simulink model "ADIODEcontrol"  (Simulink 7.3)
settings: Solver=ode4  StartTime=0.0  StopTime=tof  FixedStep=dtSim  RelTol=1e-3
InitFcn:
  | initADIODEcontrol
StopFcn:
  | plotlab
values from neighbouring files (symbols this model uses):
  Arm = -2    [initADIODEcontrol.m]
  As = -10    [initADIODEcontrol.m]
  B = 1    [initADIODEcontrol.m]
  Brm = 2    [initADIODEcontrol.m]
  dtController = dtSim    (= 0.001)    [initADIODEcontrol.m]
  epsilon = 0.05    [initADIODEcontrol.m]
  epsilontheta = 0.1    [initADIODEcontrol.m]
  GammaW = 100    [initADIODEcontrol.m]
  lambdae2 = 10    [initADIODEcontrol.m]
  nofbasis = length(xis)*length(uis)    [initADIODEcontrol.m]
  Ps = lyap(As',Q)    [initADIODEcontrol.m]
  u0 = 0    [initADIODEcontrol.m]
  W0 = zeros(nofbasis,1)    [initADIODEcontrol.m]
  Wbound = 10    [initADIODEcontrol.m]
  x0 = [0 0]'    [initADIODEcontrol.m]
  xhat0 = 0    [initADIODEcontrol.m]
  xr0 = 0    [initADIODEcontrol.m]
  xu = zeros(nofbasis,2)    [initADIODEcontrol.m]
undefined symbols (not defined in the file or in its folder): DiscIntNeverNeededParam, Intmax, Intmin
libraries: dspbuff3 x3, vrlib x1, simulink x1
settings Model: Creator=Alp  LastModifiedBy=alpmarangoz
settings SolverCC: AutoInsertRateTranBlk=on

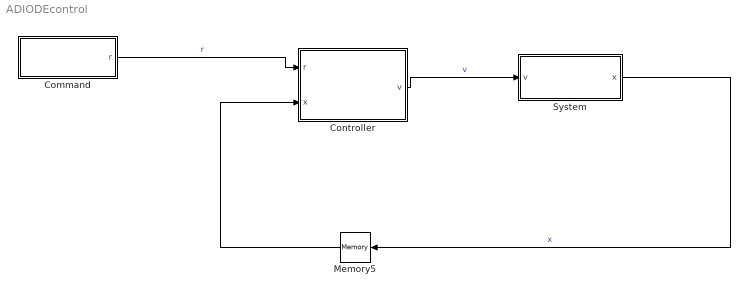
== system ADIODEcontrol ==
  Command : Subsystem  TreatAsAtomicUnit=on  SystemSampleTime=dtController
  Controller : Subsystem  TreatAsAtomicUnit=on  SystemSampleTime=dtController
  Memory5 : Memory  X0=xhat0  InheritSampleTime=on  LinearizeMemory=on  LinearizeAsDelay=on
  System : Subsystem  TreatAsAtomicUnit=on
  wires:
  Command/1(r) -> Controller/1(r)  "r"
  Controller/1(v) -> System/1(v)  "v"
  System/1(x) -> Memory5/1  "x"
  Memory5/1 -> Controller/2(x)

== system ADIODEcontrol/Command ==
  From Workspace : FromWorkspace  VariableName=rData  OutputAfterFinalValue=Setting to zero
  Reshape : Reshape  OutputDimensionality=Column vector (2-D)
  r : Outport
  wires:
  From Workspace/1 -> Reshape/1  "r"
  Reshape/1 -> r/1  "r"

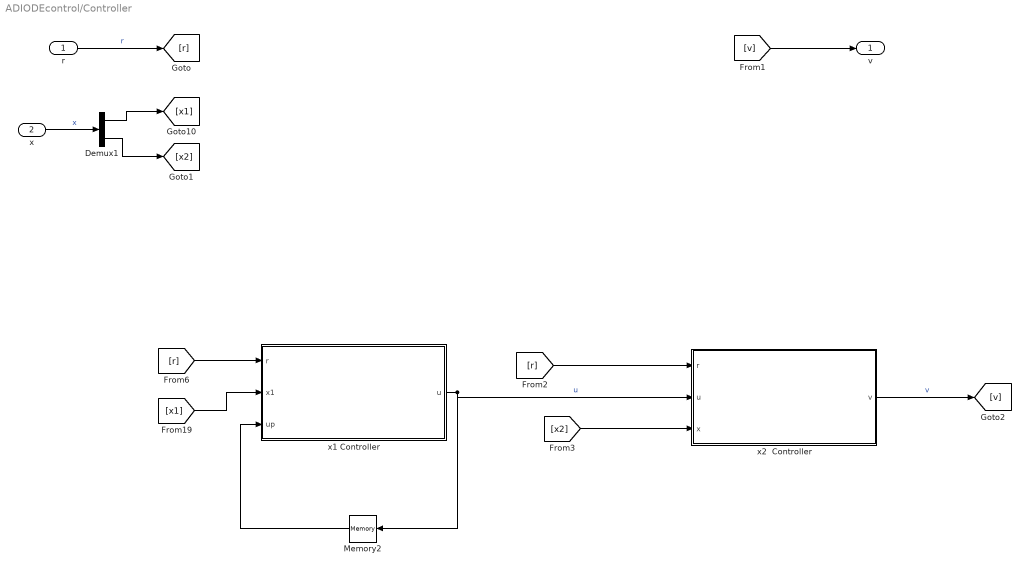
== system ADIODEcontrol/Controller ==
  r : Inport  OutDataType=fixdt(1, 16)  OutScaling=2^0
  x : Inport  Port=2  OutDataType=fixdt(1, 16)  OutScaling=2^0
  Demux1 : Demux  Outputs=2
  Memory2 : Memory  X0=u0  InheritSampleTime=on  LinearizeMemory=on  LinearizeAsDelay=on
  x1 Controller : Subsystem  TreatAsAtomicUnit=on  SystemSampleTime=dtController
  x2  Controller : Subsystem  TreatAsAtomicUnit=on  SystemSampleTime=dtController
  v : Outport  OutDataType=fixdt(1, 16)  OutScaling=2^0
  wires:
  r/1 -> [r]  "r"
  [v] -> v/1
  Demux1/1 -> [x1]
  Demux1/2 -> [x2]
  x/1 -> Demux1/1  "x"
  [r] -> x1 Controller/1(r)
  [x1] -> x1 Controller/2(x1)
  x1 Controller/1(u) -> Memory2/1, x2  Controller/2(u)  "u"
  Memory2/1 -> x1 Controller/3(up)
  [r] -> x2  Controller/1(r)
  [x2] -> x2  Controller/3(x)
  x2  Controller/1(v) -> [v]  "v"

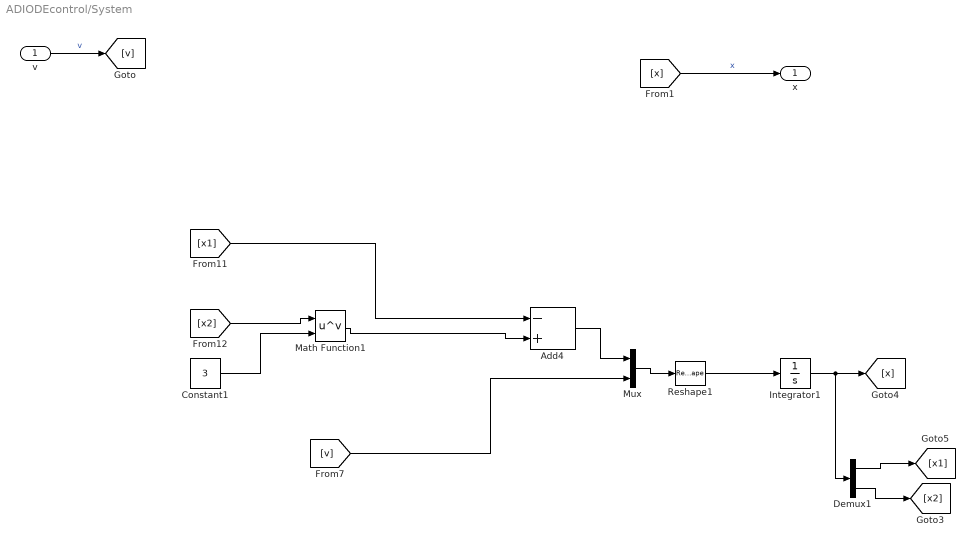
== system ADIODEcontrol/System ==
  v : Inport  OutDataType=fixdt(1, 16)  OutScaling=2^0
  Add4 : Sum  Inputs=-+  OutDataType=fixdt(1, 16)  OutScaling=2^-10
  Constant1 : Constant  Value=3  OutDataType=fixdt(1, 16)  OutScaling=2^0
  Demux1 : Demux  Outputs=2
  Integrator1 : Integrator  InitialCondition=x0
  Math Function1 : Math  Operator=pow  OutDataType=fixdt(1, 16)  OutScaling=2^0  SaturateOnIntegerOverflow=on
  Mux : Mux  Inputs=2
  Reshape1 : Reshape  OutputDimensionality=Column vector (2-D)
  x : Outport  OutDataType=fixdt(1, 16)  OutScaling=2^0
  wires:
  v/1 -> [v]  "v"
  [x] -> x/1  "x"
  [x2] -> Math Function1/1
  Constant1/1 -> Math Function1/2
  [x1] -> Add4/1
  Math Function1/1 -> Add4/2
  Integrator1/1 -> [x], Demux1/1
  Add4/1 -> Mux/1
  [v] -> Mux/2
  Mux/1 -> Reshape1/1
  Reshape1/1 -> Integrator1/1
  Demux1/1 -> [x1]
  Demux1/2 -> [x2]

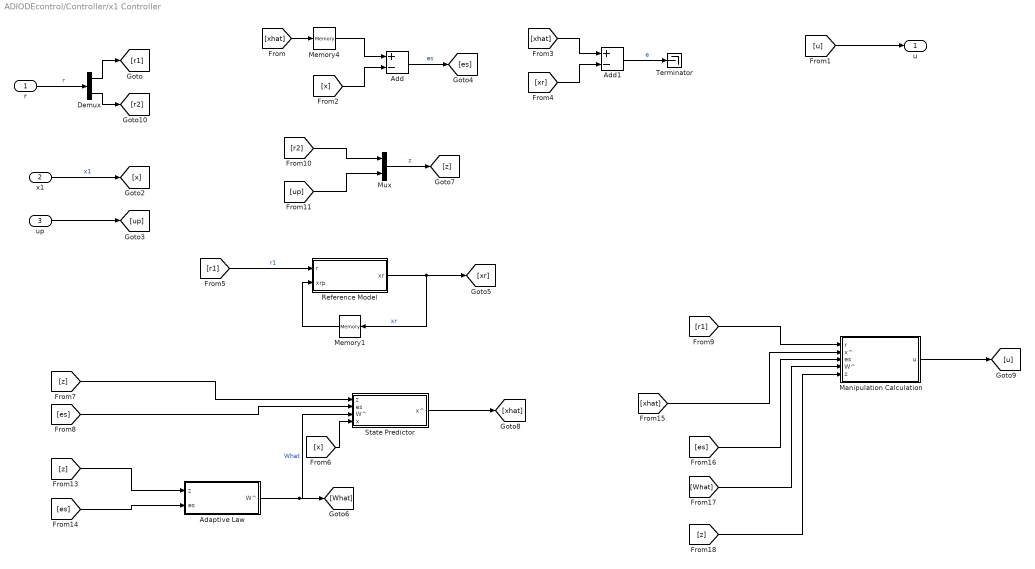
== system ADIODEcontrol/Controller/x1 Controller ==
  r : Inport  OutDataType=fixdt(1, 16)  OutScaling=2^0
  x1 : Inport  Port=2  OutDataType=fixdt(1, 16)  OutScaling=2^0
  up : Inport  Port=3  OutDataType=fixdt(1, 16)  OutScaling=2^0
  Adaptive Law : Subsystem  TreatAsAtomicUnit=on
  Add : Sum  Inputs=+-  OutDataType=fixdt(1, 16)  OutScaling=2^-10
  Add1 : Sum  Inputs=+-  OutDataType=fixdt(1, 16)  OutScaling=2^-10
  Demux : Demux  Outputs=2
  Manipulation Calculation : Subsystem  TreatAsAtomicUnit=on
  Memory1 : Memory  X0=xr0  InheritSampleTime=on  LinearizeMemory=on  LinearizeAsDelay=on
  Memory4 : Memory  X0=xhat0  InheritSampleTime=on  LinearizeMemory=on  LinearizeAsDelay=on
  Mux : Mux  Inputs=2
  Reference Model : Subsystem  TreatAsAtomicUnit=on
  State Predictor : Subsystem  TreatAsAtomicUnit=on
  Terminator : Terminator
  u : Outport  OutDataType=fixdt(1, 16)  OutScaling=2^0
  wires:
  [u] -> u/1
  x1/1 -> [x]  "x1"
  up/1 -> [up]
  [xhat] -> Memory4/1
  [x] -> Add/2
  [xhat] -> Add1/1
  [xr] -> Add1/2
  Add/1 -> [es]  "es"
  Add1/1 -> Terminator/1  "e"
  Reference Model/1(xr) -> [xr], Memory1/1  "xr"
  [r1] -> Reference Model/1(r)  "r1"
  Memory4/1 -> Add/1
  [z] -> Adaptive Law/1(z)
  [es] -> Adaptive Law/2(es)
  Adaptive Law/1(W^) -> State Predictor/3(W^), [What]  "What"
  [z] -> State Predictor/1(z)
  [es] -> State Predictor/2(es)
  State Predictor/1(x^) -> [xhat]
  [r1] -> Manipulation Calculation/1(r)
  [xhat] -> Manipulation Calculation/2(x^)
  [es] -> Manipulation Calculation/3(es)
  [What] -> Manipulation Calculation/4(W^)
  [z] -> Manipulation Calculation/5(z)
  Manipulation Calculation/1(u) -> [u]
  Memory1/1 -> Reference Model/2(xrp)
  [r2] -> Mux/1
  [up] -> Mux/2
  Mux/1 -> [z]  "z"
  [x] -> State Predictor/4(x)
  r/1 -> Demux/1  "r"
  Demux/1 -> [r1]
  Demux/2 -> [r2]

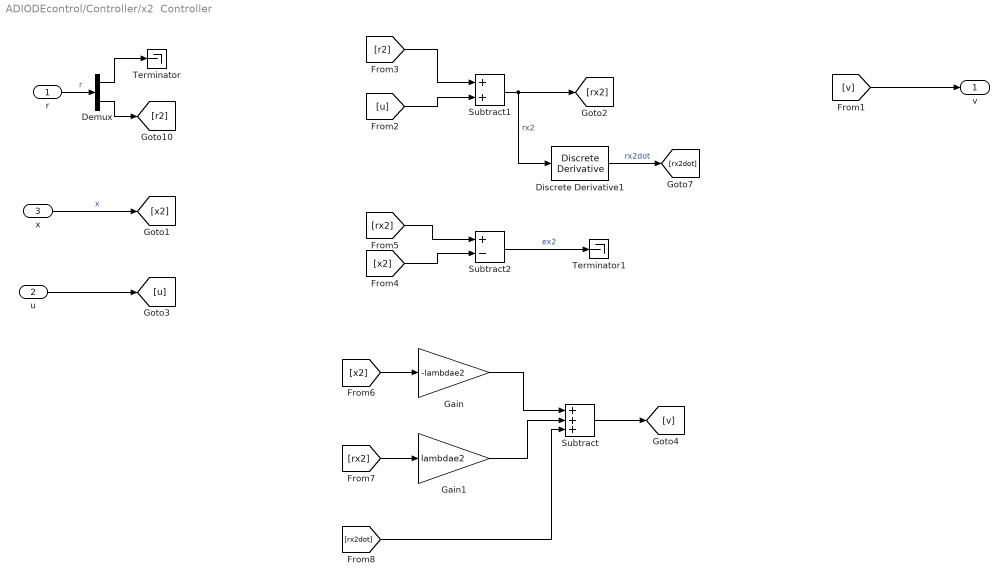
== system ADIODEcontrol/Controller/x2  Controller ==
  r : Inport  OutDataType=fixdt(1, 16)  OutScaling=2^0
  u : Inport  Port=2  OutDataType=fixdt(1, 16)  OutScaling=2^0
  x : Inport  Port=3  OutDataType=fixdt(1, 16)  OutScaling=2^0
  Demux : Demux  Outputs=2
  Discrete Derivative1 : simulink/Discrete/Discrete Derivative  SystemSampleTime=-1  gainval=1.0  ICPrevScaledInput=0.0  OutMin=[]  OutMax=[]  OutDataType=fixdt(1, 16)  OutScaling=2^-10  DoSatur=off
  Gain : Gain  Gain=-lambdae2  ParameterDataType=fixdt(1, 16)  ParameterScaling=2^0  OutDataType=fixdt(1, 16)  OutScaling=2^0
  Gain1 : Gain  Gain=lambdae2  ParameterDataType=fixdt(1, 16)  ParameterScaling=2^0  OutDataType=fixdt(1, 16)  OutScaling=2^0
  Subtract : Sum  Inputs=+++  OutDataType=fixdt(1, 16)  OutScaling=2^-10
  Subtract1 : Sum  OutDataType=fixdt(1, 16)  OutScaling=2^-10
  Subtract2 : Sum  Inputs=+-  OutDataType=fixdt(1, 16)  OutScaling=2^-10
  Terminator : Terminator
  Terminator1 : Terminator
  v : Outport  OutDataType=fixdt(1, 16)  OutScaling=2^0
  wires:
  Demux/2 -> [r2]
  Demux/1 -> Terminator/1
  r/1 -> Demux/1  "r"
  u/1 -> [u]
  [v] -> v/1
  x/1 -> [x2]  "x"
  [x2] -> Gain/1
  [rx2] -> Gain1/1
  Gain/1 -> Subtract/1
  Gain1/1 -> Subtract/2
  [r2] -> Subtract1/1
  [u] -> Subtract1/2
  Subtract1/1 -> [rx2], Discrete Derivative1/1  "rx2"
  Subtract/1 -> [v]
  [x2] -> Subtract2/2
  Subtract2/1 -> Terminator1/1  "ex2"
  [rx2] -> Subtract2/1
  Discrete Derivative1/1 -> [rx2dot]  "rx2dot"
  [rx2dot] -> Subtract/3

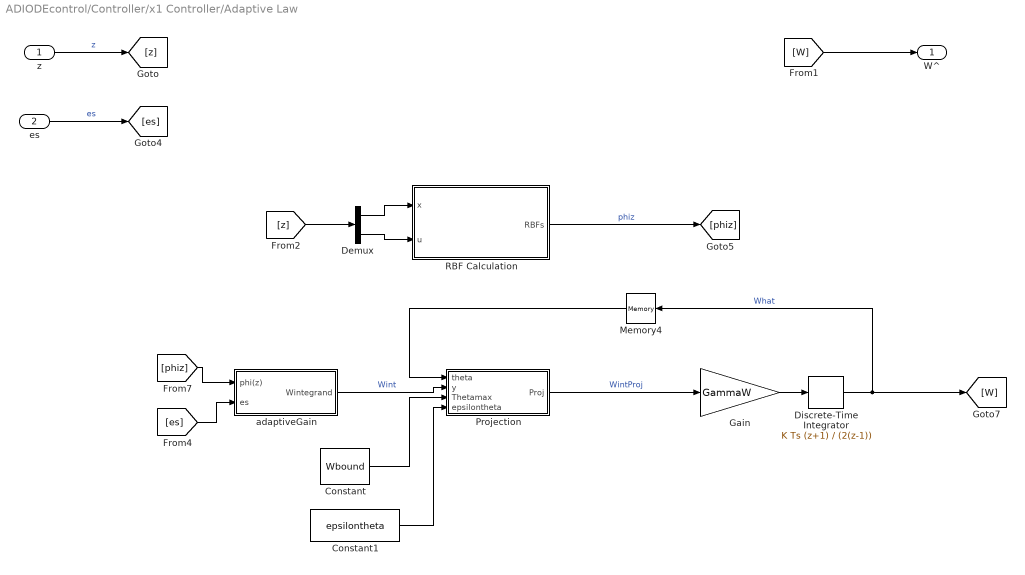
== system ADIODEcontrol/Controller/x1 Controller/Adaptive Law ==
  z : Inport  OutDataType=fixdt(1, 16)  OutScaling=2^0
  es : Inport  Port=2  OutDataType=fixdt(1, 16)  OutScaling=2^0
  Constant : Constant  Value=Wbound  OutDataType=fixdt(1, 16)  OutScaling=2^0
  Constant1 : Constant  Value=epsilontheta  OutDataType=fixdt(1, 16)  OutScaling=2^0
  Demux : Demux  Outputs=2
  Discrete-Time Integrator : DiscreteIntegrator  IntegratorMethod=Integration: Trapezoidal  InitialCondition=W0  SampleTime=-1  OutDataType=fixdt(1, 16)  OutScaling=2^0  LimitOutput=on  UpperSaturationLimit=Wbound  LowerSaturationLimit=-Wbound  ICPrevOutput=DiscIntNeverNeededParam  ICPrevScaledInput=DiscIntNeverNeededParam
  Gain : Gain  Gain=GammaW  ParameterDataType=fixdt(1, 16)  ParameterScaling=2^0  OutDataType=fixdt(1, 16)  OutScaling=2^0
  Memory4 : Memory  X0=W0  InheritSampleTime=on  LinearizeMemory=on  LinearizeAsDelay=on
  Projection : Subsystem  TreatAsAtomicUnit=on
  RBF Calculation : Subsystem  TreatAsAtomicUnit=on
  adaptiveGain : Subsystem  TreatAsAtomicUnit=on
  W^ : Outport  OutDataType=fixdt(1, 16)  OutScaling=2^0
  wires:
  z/1 -> [z]  "z"
  es/1 -> [es]  "es"
  [es] -> adaptiveGain/2(es)
  [phiz] -> adaptiveGain/1(phi(z))
  [W] -> W^/1
  Discrete-Time Integrator/1 -> [W], Memory4/1  "What"
  Gain/1 -> Discrete-Time Integrator/1
  RBF Calculation/1(RBFs) -> [phiz]  "phiz"
  [z] -> Demux/1
  Demux/1 -> RBF Calculation/1(x)
  Demux/2 -> RBF Calculation/2(u)
  Projection/1(Proj) -> Gain/1  "WintProj"
  adaptiveGain/1(Wintegrand) -> Projection/2(y)  "Wint"
  Memory4/1 -> Projection/1(theta)
  Constant/1 -> Projection/3(Thetamax)
  Constant1/1 -> Projection/4(epsilontheta)

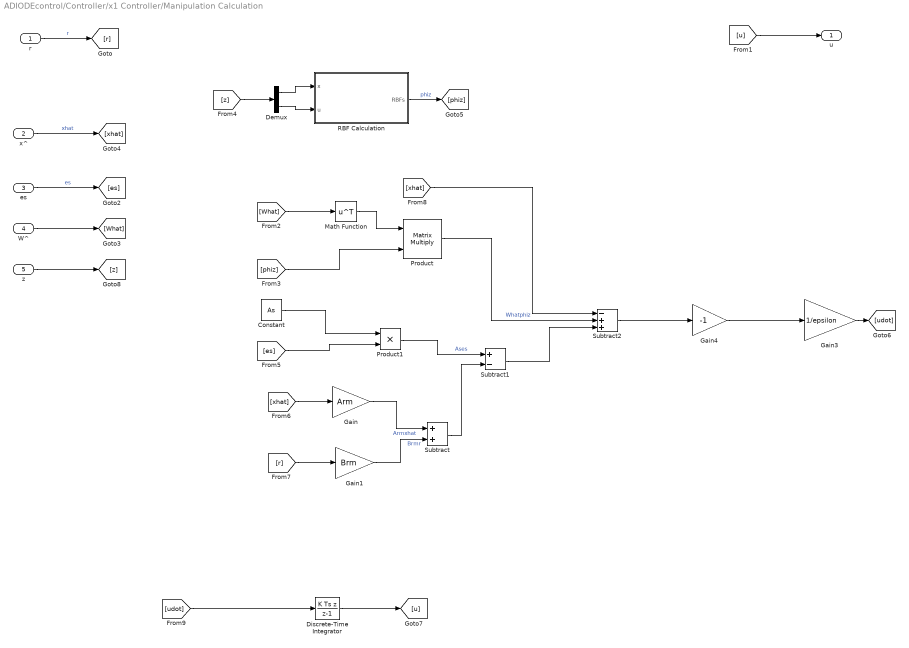
== system ADIODEcontrol/Controller/x1 Controller/Manipulation Calculation ==
  r : Inport  OutDataType=fixdt(1, 16)  OutScaling=2^0
  x^ : Inport  Port=2  OutDataType=fixdt(1, 16)  OutScaling=2^0
  es : Inport  Port=3  OutDataType=fixdt(1, 16)  OutScaling=2^0
  W^ : Inport  Port=4  OutDataType=fixdt(1, 16)  OutScaling=2^0
  z : Inport  Port=5  OutDataType=fixdt(1, 16)  OutScaling=2^0
  Constant : Constant  Value=As  OutDataType=fixdt(1, 16)  OutScaling=2^0
  Demux : Demux  Outputs=2
  Discrete-Time Integrator : DiscreteIntegrator  IntegratorMethod=Integration: Backward Euler  InitialCondition=u0  InitialConditionMode=State only (most efficient)  SampleTime=-1  OutDataType=fixdt(1, 16)  OutScaling=2^0  UpperSaturationLimit=Intmax  LowerSaturationLimit=Intmin  ICPrevOutput=DiscIntNeverNeededParam  ICPrevScaledInput=DiscIntNeverNeededParam
  Gain : Gain  Gain=Arm  ParameterDataType=fixdt(1, 16)  ParameterScaling=2^0  OutDataType=fixdt(1, 16)  OutScaling=2^0
  Gain1 : Gain  Gain=Brm  ParameterDataType=fixdt(1, 16)  ParameterScaling=2^0  OutDataType=fixdt(1, 16)  OutScaling=2^0
  Gain3 : Gain  Gain=1/epsilon  ParameterDataType=fixdt(1, 16)  ParameterScaling=2^0  OutDataType=fixdt(1, 16)  OutScaling=2^0
  Gain4 : Gain  Gain=-1  ParameterDataType=fixdt(1, 16)  ParameterScaling=2^0  OutDataType=fixdt(1, 16)  OutScaling=2^0
  Math Function : Math  Operator=transpose  OutDataType=fixdt(1, 16)  OutScaling=2^0  SaturateOnIntegerOverflow=on
  Product : Product  Multiplication=Matrix(*)  OutDataType=fixdt(1, 16)  OutScaling=2^0  RndMeth=Zero
  Product1 : Product  OutDataType=fixdt(1, 16)  OutScaling=2^0  RndMeth=Zero
  RBF Calculation : Subsystem  TreatAsAtomicUnit=on
  Subtract : Sum  OutDataType=fixdt(1, 16)  OutScaling=2^-10
  Subtract1 : Sum  Inputs=+-  OutDataType=fixdt(1, 16)  OutScaling=2^-10
  Subtract2 : Sum  Inputs=-++  OutDataType=fixdt(1, 16)  OutScaling=2^-10
  u : Outport  OutDataType=fixdt(1, 16)  OutScaling=2^0
  wires:
  r/1 -> [r]  "r"
  [u] -> u/1
  x^/1 -> [xhat]  "xhat"
  es/1 -> [es]  "es"
  W^/1 -> [What]
  [What] -> Math Function/1
  Math Function/1 -> Product/1
  [phiz] -> Product/2
  Constant/1 -> Product1/1
  [xhat] -> Gain/1
  [r] -> Gain1/1
  Gain3/1 -> [udot]
  z/1 -> [z]
  [es] -> Product1/2
  RBF Calculation/1(RBFs) -> [phiz]  "phiz"
  [z] -> Demux/1
  Demux/1 -> RBF Calculation/1(x)
  Demux/2 -> RBF Calculation/2(u)
  [udot] -> Discrete-Time Integrator/1
  Discrete-Time Integrator/1 -> [u]
  Gain4/1 -> Gain3/1
  Gain/1 -> Subtract/1  "Armxhat"
  Gain1/1 -> Subtract/2  "Brmr"
  Product1/1 -> Subtract1/1  "Ases"
  Subtract/1 -> Subtract1/2
  Subtract2/1 -> Gain4/1
  [xhat] -> Subtract2/1
  Product/1 -> Subtract2/2  "Whatphiz"
  Subtract1/1 -> Subtract2/3

== system ADIODEcontrol/Controller/x1 Controller/Reference Model ==
  r : Inport  OutDataType=fixdt(1, 16)  OutScaling=2^0
  xrp : Inport  Port=2  OutDataType=fixdt(1, 16)  OutScaling=2^0
  Add1 : Sum  OutDataType=fixdt(1, 16)  OutScaling=2^-10
  Discrete-Time Integrator : DiscreteIntegrator  IntegratorMethod=Integration: Backward Euler  InitialCondition=xr0  InitialConditionMode=State only (most efficient)  SampleTime=-1  OutDataType=fixdt(1, 16)  OutScaling=2^0  UpperSaturationLimit=Intmax  LowerSaturationLimit=Intmin  ICPrevOutput=DiscIntNeverNeededParam  ICPrevScaledInput=DiscIntNeverNeededParam
  Gain1 : Gain  Gain=Arm  Multiplication=Matrix(K*u)  ParameterDataType=fixdt(1, 16)  ParameterScaling=2^0  OutDataType=fixdt(1, 16)  OutScaling=2^0
  Gain2 : Gain  Gain=Brm  Multiplication=Matrix(K*u)  ParameterDataType=fixdt(1, 16)  ParameterScaling=2^0  OutDataType=fixdt(1, 16)  OutScaling=2^0
  Reshape : Reshape  OutputDimensionality=Column vector (2-D)
  xr : Outport  OutDataType=fixdt(1, 16)  OutScaling=2^0
  wires:
  [xrp] -> Gain1/1
  r/1 -> [u]  "r"
  [u] -> Gain2/1
  Gain1/1 -> Add1/1
  Gain2/1 -> Add1/2
  Add1/1 -> Reshape/1  "xrmdot"
  Reshape/1 -> Discrete-Time Integrator/1
  Discrete-Time Integrator/1 -> xr/1  "xr"
  xrp/1 -> [xrp]

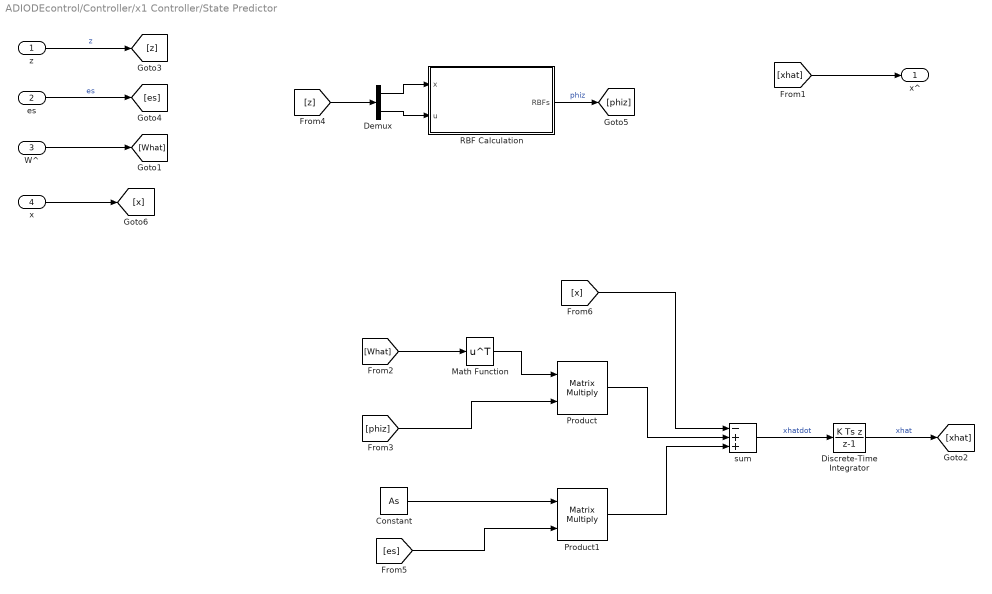
== system ADIODEcontrol/Controller/x1 Controller/State Predictor ==
  z : Inport  OutDataType=fixdt(1, 16)  OutScaling=2^0
  es : Inport  Port=2  OutDataType=fixdt(1, 16)  OutScaling=2^0
  W^ : Inport  Port=3  OutDataType=fixdt(1, 16)  OutScaling=2^0
  x : Inport  Port=4  OutDataType=fixdt(1, 16)  OutScaling=2^0
  Constant : Constant  Value=As  OutDataType=fixdt(1, 16)  OutScaling=2^0
  Demux : Demux  Outputs=2
  Discrete-Time Integrator : DiscreteIntegrator  IntegratorMethod=Integration: Backward Euler  InitialCondition=xhat0  InitialConditionMode=State only (most efficient)  SampleTime=-1  OutDataType=fixdt(1, 16)  OutScaling=2^0  UpperSaturationLimit=Intmax  LowerSaturationLimit=Intmin  ICPrevOutput=DiscIntNeverNeededParam  ICPrevScaledInput=DiscIntNeverNeededParam
  Math Function : Math  Operator=transpose  OutDataType=fixdt(1, 16)  OutScaling=2^0  SaturateOnIntegerOverflow=on
  Product : Product  Multiplication=Matrix(*)  OutDataType=fixdt(1, 16)  OutScaling=2^0  RndMeth=Zero
  Product1 : Product  Multiplication=Matrix(*)  OutDataType=fixdt(1, 16)  OutScaling=2^0  RndMeth=Zero
  RBF Calculation : Subsystem  TreatAsAtomicUnit=on
  sum : Sum  Inputs=-++  OutDataType=fixdt(1, 16)  OutScaling=2^-10
  x^ : Outport  OutDataType=fixdt(1, 16)  OutScaling=2^0
  wires:
  W^/1 -> [What]
  es/1 -> [es]  "es"
  [What] -> Math Function/1
  Math Function/1 -> Product/1
  [phiz] -> Product/2
  Constant/1 -> Product1/1
  [es] -> Product1/2
  sum/1 -> Discrete-Time Integrator/1  "xhatdot"
  Discrete-Time Integrator/1 -> [xhat]  "xhat"
  z/1 -> [z]  "z"
  [xhat] -> x^/1
  RBF Calculation/1(RBFs) -> [phiz]  "phiz"
  [z] -> Demux/1
  Demux/1 -> RBF Calculation/1(x)
  Demux/2 -> RBF Calculation/2(u)
  x/1 -> [x]
  [x] -> sum/1
  Product/1 -> sum/2
  Product1/1 -> sum/3

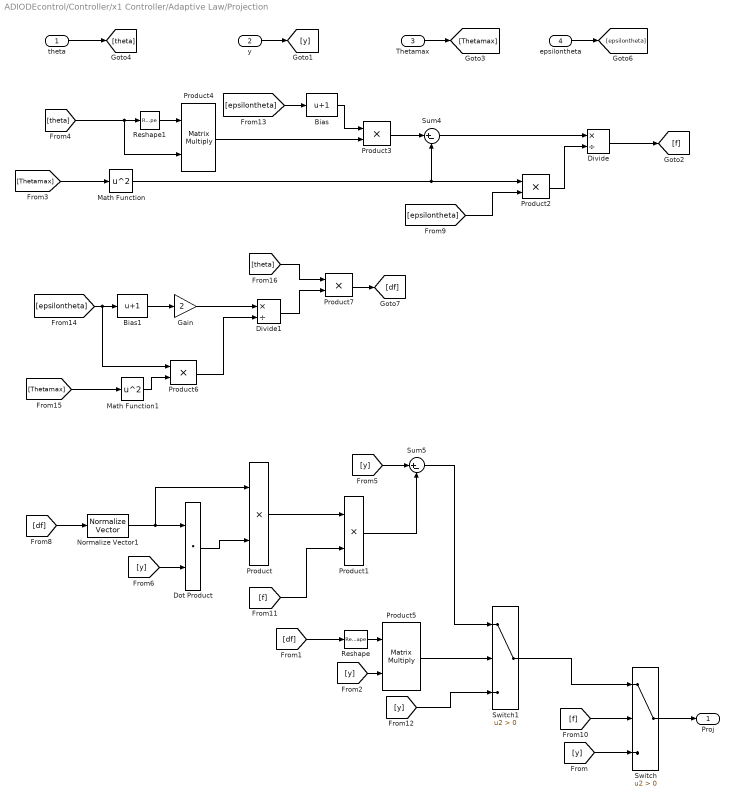
== system ADIODEcontrol/Controller/x1 Controller/Adaptive Law/Projection ==
  theta : Inport  OutDataType=sfix(16)  OutScaling=2^0
  y : Inport  Port=2  OutDataType=sfix(16)  OutScaling=2^0
  Thetamax : Inport  Port=3  OutDataType=sfix(16)  OutScaling=2^0
  epsilontheta : Inport  Port=4  OutDataType=sfix(16)  OutScaling=2^0
  Bias : Bias  Bias=1
  Bias1 : Bias  Bias=1
  Divide : Product  Inputs=*/  OutDataType=fixdt(1, 16)  OutScaling=2^-10
  Divide1 : Product  Inputs=*/  OutDataType=fixdt(1, 16)  OutScaling=2^-10
  Dot Product : DotProduct  OutDataType=fixdt(1, 16)  OutScaling=2^-10  InputSameDT=on  OutDataTypeStr=Inherit: Inherit via internal rule
  Gain : Gain  Gain=2  ParameterDataType=fixdt(1, 16)  ParameterScaling=2^0  OutDataType=fixdt(1, 16)  OutScaling=2^0
  Math Function : Math  Operator=square  OutDataType=fixdt(1, 16)  OutScaling=2^0  SaturateOnIntegerOverflow=on
  Math Function1 : Math  Operator=square  OutDataType=fixdt(1, 16)  OutScaling=2^0  SaturateOnIntegerOverflow=on
  Normalize Vector1 : vrlib/Utilities/Normalize Vector  SystemSampleTime=-1  maxzero=0
  Product{,1..3,6..7} (6 alike) : Product  OutDataType=fixdt(1, 16)  OutScaling=2^0  RndMeth=Zero
  Product4 : Product  Multiplication=Matrix(*)  OutDataType=sfix(16)  OutScaling=2^0  RndMeth=Zero
  Product5 : Product  Multiplication=Matrix(*)  OutDataType=sfix(16)  OutScaling=2^0  RndMeth=Zero
  Reshape : Reshape  OutputDimensionality=Row vector (2-D)
  Reshape1 : Reshape  OutputDimensionality=Row vector (2-D)
  Sum4 : Sum  Inputs=|+-  OutDataType=sfix(16)  OutScaling=2^0
  Sum5 : Sum  Inputs=|+-  OutDataType=sfix(16)  OutScaling=2^0
  Switch : Switch  Criteria=u2 > Threshold  OutDataType=sfix(16)  OutScaling=2^0
  Switch1 : Switch  Criteria=u2 > Threshold  OutDataType=sfix(16)  OutScaling=2^0
  Proj : Outport  OutDataType=sfix(16)  OutScaling=2^0
  wires:
  [f] -> Switch/2
  y/1 -> [y]
  Switch/1 -> Proj/1
  Product5/1 -> Switch1/2
  [y] -> Product5/2
  Sum4/1 -> Divide/1
  Math Function/1 -> Sum4/2, Product2/1
  Product4/1 -> Product3/2
  [theta] -> Reshape1/1, Product4/2
  [df] -> Reshape/1
  Reshape/1 -> Product5/1
  Reshape1/1 -> Product4/1
  theta/1 -> [theta]
  [y] -> Switch/3
  Switch1/1 -> Switch/1
  [y] -> Sum5/1
  Product/1 -> Product1/1
  [y] -> Switch1/3
  Product1/1 -> Sum5/2
  Sum5/1 -> Switch1/1
  [f] -> Product1/2
  [df] -> Normalize Vector1/1
  Normalize Vector1/1 -> Dot Product/1, Product/1
  [y] -> Dot Product/2
  Dot Product/1 -> Product/2
  Thetamax/1 -> [Thetamax]
  [Thetamax] -> Math Function/1
  epsilontheta/1 -> [epsilontheta]
  [epsilontheta] -> Product2/2
  Product2/1 -> Divide/2
  Divide/1 -> [f]
  Product3/1 -> Sum4/1
  Bias/1 -> Product3/1
  [epsilontheta] -> Bias/1
  [epsilontheta] -> Bias1/1, Product6/1
  Bias1/1 -> Gain/1
  Gain/1 -> Divide1/1
  [Thetamax] -> Math Function1/1
  Math Function1/1 -> Product6/2
  Product6/1 -> Divide1/2
  Product7/1 -> [df]
  [theta] -> Product7/1
  Divide1/1 -> Product7/2

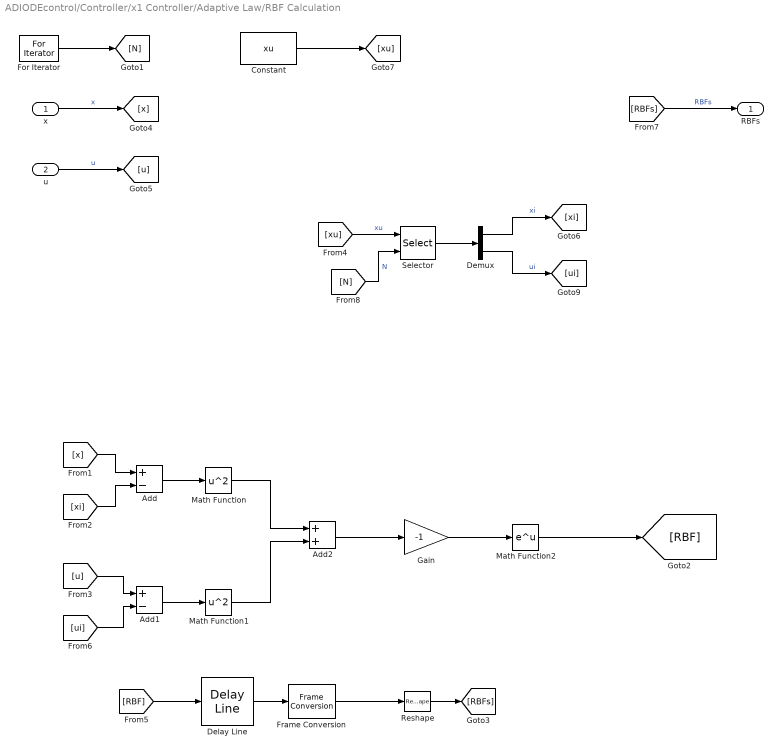
== system ADIODEcontrol/Controller/x1 Controller/Adaptive Law/RBF Calculation ==
  x : Inport  OutDataType=fixdt(1, 16)  OutScaling=2^0
  u : Inport  Port=2  OutDataType=fixdt(1, 16)  OutScaling=2^0
  Add : Sum  Inputs=+-  OutDataType=fixdt(1, 16)  OutScaling=2^-10
  Add1 : Sum  Inputs=+-  OutDataType=fixdt(1, 16)  OutScaling=2^-10
  Add2 : Sum  OutDataType=fixdt(1, 16)  OutScaling=2^-10
  Constant : Constant  Value=xu  VectorParams1D=off  OutDataType=fixdt(1, 16)  OutScaling=2^0
  Delay Line : dspbuff3/Delay Line  siz=nofbasis  ic=zeros(nofbasis,1)  directfeed=on  enable_output=off  hold_output=off
  Demux : Demux  Outputs=2
  For Iterator : ForIterator  IterationLimit=nofbasis
  Frame Conversion : FrameConversion  OutFrame=Sample-based
  Gain : Gain  Gain=-1  ParameterDataType=fixdt(1, 16)  ParameterScaling=2^0  OutDataType=fixdt(1, 16)  OutScaling=2^0
  Math Function : Math  Operator=square  OutDataType=fixdt(1, 16)  OutScaling=2^0  SaturateOnIntegerOverflow=on
  Math Function1 : Math  Operator=square  OutDataType=fixdt(1, 16)  OutScaling=2^0  SaturateOnIntegerOverflow=on
  Math Function2 : Math  OutDataType=fixdt(1, 16)  OutScaling=2^0  SaturateOnIntegerOverflow=on
  Reshape : Reshape  OutputDimensionality=Column vector (2-D)
  Selector : Selector  NumberOfDimensions=2  IndexOptions=Index vector (port),Select all  Indices=[1 3],1  OutputSizes=1,1
  RBFs : Outport  OutDataType=fixdt(1, 16)  OutScaling=2^0
  wires:
  For Iterator/1 -> [N]
  [RBF] -> Delay Line/1
  Delay Line/1 -> Frame Conversion/1
  [RBFs] -> RBFs/1  "RBFs"
  Frame Conversion/1 -> Reshape/1
  x/1 -> [x]  "x"
  u/1 -> [u]  "u"
  [xu] -> Selector/1  "xu"
  [N] -> Selector/2  "N"
  [x] -> Add/1
  [xi] -> Add/2
  Add/1 -> Math Function/1
  [u] -> Add1/1
  [ui] -> Add1/2
  Add1/1 -> Math Function1/1
  Math Function/1 -> Add2/1
  Math Function1/1 -> Add2/2
  Add2/1 -> Gain/1
  Gain/1 -> Math Function2/1
  Math Function2/1 -> [RBF]
  Reshape/1 -> [RBFs]
  Constant/1 -> [xu]
  Selector/1 -> Demux/1
  Demux/1 -> [xi]  "xi"
  Demux/2 -> [ui]  "ui"

== system ADIODEcontrol/Controller/x1 Controller/Adaptive Law/adaptiveGain ==
  phi(z) : Inport  OutDataType=fixdt(1, 16)  OutScaling=2^0
  es : Inport  Port=2  OutDataType=fixdt(1, 16)  OutScaling=2^0
  Gain1 : Gain  Gain=-1  ParameterDataType=fixdt(1, 16)  ParameterScaling=2^0  OutDataType=fixdt(1, 16)  OutScaling=2^0
  Math Function : Math  Operator=transpose  OutDataType=sfix(16)  OutScaling=2^0  SaturateOnIntegerOverflow=on
  P : Constant  Value=Ps  VectorParams1D=off  OutDataType=fixdt(1, 16)  OutScaling=2^0
  Product1 : Product  Multiplication=Matrix(*)  OutDataType=fixdt(1, 16)  OutScaling=2^0  RndMeth=Zero
  Product3 : Product  Multiplication=Matrix(*)  OutDataType=fixdt(1, 16)  OutScaling=2^0  RndMeth=Zero
  Product5 : Product  Multiplication=Matrix(*)  OutDataType=fixdt(1, 16)  OutScaling=2^0  RndMeth=Zero
  b : Constant  Value=B  VectorParams1D=off  OutDataType=fixdt(1, 16)  OutScaling=2^0
  Wintegrand : Outport  OutDataType=fixdt(1, 16)  OutScaling=2^0
  wires:
  P/1 -> Product5/1
  b/1 -> Product5/2
  es/1 -> Math Function/1
  Math Function/1 -> Product1/1
  Product5/1 -> Product1/2
  phi(z)/1 -> Gain1/1
  Product1/1 -> Product3/2
  Product3/1 -> Wintegrand/1
  Gain1/1 -> Product3/1

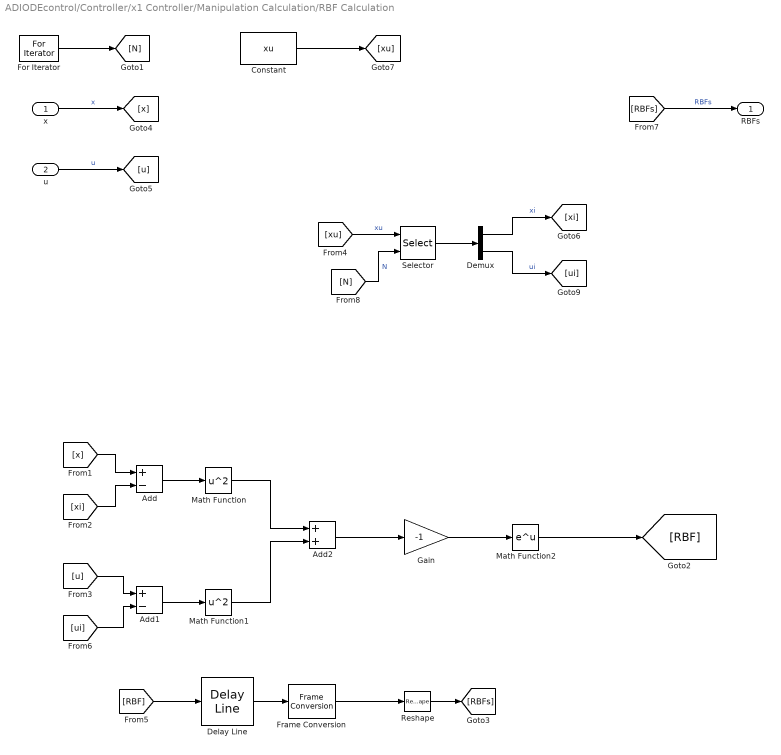
== system ADIODEcontrol/Controller/x1 Controller/Manipulation Calculation/RBF Calculation ==
  x : Inport  OutDataType=fixdt(1, 16)  OutScaling=2^0
  u : Inport  Port=2  OutDataType=fixdt(1, 16)  OutScaling=2^0
  Add : Sum  Inputs=+-  OutDataType=fixdt(1, 16)  OutScaling=2^-10
  Add1 : Sum  Inputs=+-  OutDataType=fixdt(1, 16)  OutScaling=2^-10
  Add2 : Sum  OutDataType=fixdt(1, 16)  OutScaling=2^-10
  Constant : Constant  Value=xu  VectorParams1D=off  OutDataType=fixdt(1, 16)  OutScaling=2^0
  Delay Line : dspbuff3/Delay Line  siz=nofbasis  ic=zeros(nofbasis,1)  directfeed=on  enable_output=off  hold_output=off
  Demux : Demux  Outputs=2
  For Iterator : ForIterator  IterationLimit=nofbasis
  Frame Conversion : FrameConversion  OutFrame=Sample-based
  Gain : Gain  Gain=-1  ParameterDataType=fixdt(1, 16)  ParameterScaling=2^0  OutDataType=fixdt(1, 16)  OutScaling=2^0
  Math Function : Math  Operator=square  OutDataType=fixdt(1, 16)  OutScaling=2^0  SaturateOnIntegerOverflow=on
  Math Function1 : Math  Operator=square  OutDataType=fixdt(1, 16)  OutScaling=2^0  SaturateOnIntegerOverflow=on
  Math Function2 : Math  OutDataType=fixdt(1, 16)  OutScaling=2^0  SaturateOnIntegerOverflow=on
  Reshape : Reshape  OutputDimensionality=Column vector (2-D)
  Selector : Selector  NumberOfDimensions=2  IndexOptions=Index vector (port),Select all  Indices=[1 3],1  OutputSizes=1,1
  RBFs : Outport  OutDataType=fixdt(1, 16)  OutScaling=2^0
  wires:
  For Iterator/1 -> [N]
  [RBF] -> Delay Line/1
  Delay Line/1 -> Frame Conversion/1
  [RBFs] -> RBFs/1  "RBFs"
  Frame Conversion/1 -> Reshape/1
  x/1 -> [x]  "x"
  u/1 -> [u]  "u"
  [xu] -> Selector/1  "xu"
  [N] -> Selector/2  "N"
  [x] -> Add/1
  [xi] -> Add/2
  Add/1 -> Math Function/1
  [u] -> Add1/1
  [ui] -> Add1/2
  Add1/1 -> Math Function1/1
  Math Function/1 -> Add2/1
  Math Function1/1 -> Add2/2
  Add2/1 -> Gain/1
  Gain/1 -> Math Function2/1
  Math Function2/1 -> [RBF]
  Reshape/1 -> [RBFs]
  Constant/1 -> [xu]
  Selector/1 -> Demux/1
  Demux/1 -> [xi]  "xi"
  Demux/2 -> [ui]  "ui"

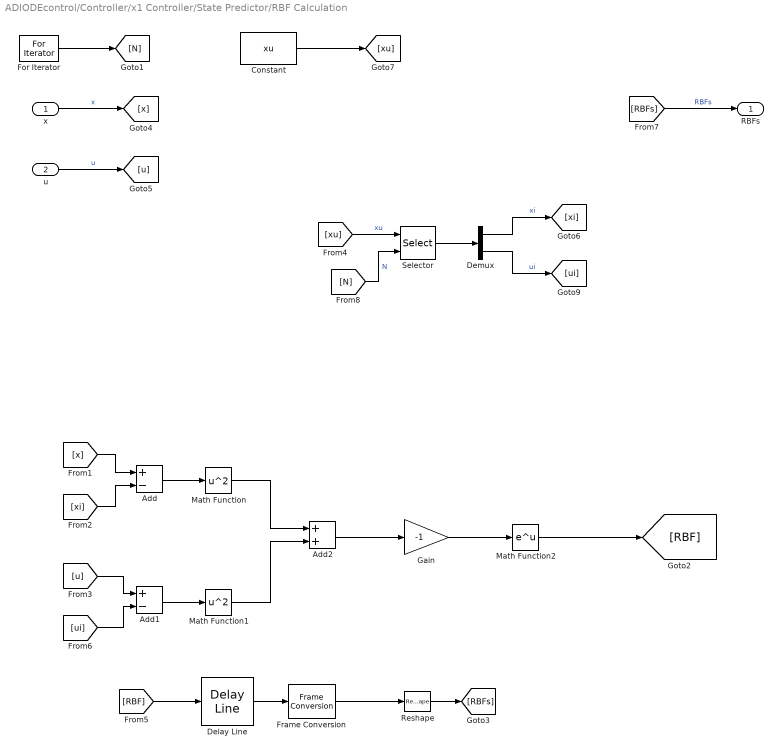
== system ADIODEcontrol/Controller/x1 Controller/State Predictor/RBF Calculation ==
  x : Inport  OutDataType=fixdt(1, 16)  OutScaling=2^0
  u : Inport  Port=2  OutDataType=fixdt(1, 16)  OutScaling=2^0
  Add : Sum  Inputs=+-  OutDataType=fixdt(1, 16)  OutScaling=2^-10
  Add1 : Sum  Inputs=+-  OutDataType=fixdt(1, 16)  OutScaling=2^-10
  Add2 : Sum  OutDataType=fixdt(1, 16)  OutScaling=2^-10
  Constant : Constant  Value=xu  VectorParams1D=off  OutDataType=fixdt(1, 16)  OutScaling=2^0
  Delay Line : dspbuff3/Delay Line  siz=nofbasis  ic=zeros(nofbasis,1)  directfeed=on  enable_output=off  hold_output=off
  Demux : Demux  Outputs=2
  For Iterator : ForIterator  IterationLimit=nofbasis
  Frame Conversion : FrameConversion  OutFrame=Sample-based
  Gain : Gain  Gain=-1  ParameterDataType=fixdt(1, 16)  ParameterScaling=2^0  OutDataType=fixdt(1, 16)  OutScaling=2^0
  Math Function : Math  Operator=square  OutDataType=fixdt(1, 16)  OutScaling=2^0  SaturateOnIntegerOverflow=on
  Math Function1 : Math  Operator=square  OutDataType=fixdt(1, 16)  OutScaling=2^0  SaturateOnIntegerOverflow=on
  Math Function2 : Math  OutDataType=fixdt(1, 16)  OutScaling=2^0  SaturateOnIntegerOverflow=on
  Reshape : Reshape  OutputDimensionality=Column vector (2-D)
  Selector : Selector  NumberOfDimensions=2  IndexOptions=Index vector (port),Select all  Indices=[1 3],1  OutputSizes=1,1
  RBFs : Outport  OutDataType=fixdt(1, 16)  OutScaling=2^0
  wires:
  For Iterator/1 -> [N]
  [RBF] -> Delay Line/1
  Delay Line/1 -> Frame Conversion/1
  [RBFs] -> RBFs/1  "RBFs"
  Frame Conversion/1 -> Reshape/1
  x/1 -> [x]  "x"
  u/1 -> [u]  "u"
  [xu] -> Selector/1  "xu"
  [N] -> Selector/2  "N"
  [x] -> Add/1
  [xi] -> Add/2
  Add/1 -> Math Function/1
  [u] -> Add1/1
  [ui] -> Add1/2
  Add1/1 -> Math Function1/1
  Math Function/1 -> Add2/1
  Math Function1/1 -> Add2/2
  Add2/1 -> Gain/1
  Gain/1 -> Math Function2/1
  Math Function2/1 -> [RBF]
  Reshape/1 -> [RBFs]
  Constant/1 -> [xu]
  Selector/1 -> Demux/1
  Demux/1 -> [xi]  "xi"
  Demux/2 -> [ui]  "ui"
